simulink model "usrp_fm_amfm"  (R2014b)
settings: Solver=ode45  StartTime=0.0  StopTime=inf  RelTol=1e-3
PreLoadFcn:
  | %%%%%%%%%%%%%%%%%%%%%%%%%%%%%%%%%%%%%%%%%%%%%%%%%%%%%%%%%%%%%%%%%%%%%%%%%%%
  | % check to see if Simulink library folder is missing from the MATLAB path %
  | %%%%%%%%%%%%%%%%%%%%%%%%%%%%%%%%%%%%%%%%%%%%%%%%%%%%%%%%%%%%%%%%%%%%%%%%%%%
  | if isempty(strfind(path, 'rtlsdr_book_library'))
  | 
  |     % create error window
  |     fig_error = figure(...
  |         'Name', 'Error: RTL-SDR Book Library',...
  |         'Toolbar','none',...
  |         'MenuBar','none',...
  |         'NumberTitle','off',...
  |         'Resize','off',...
  |         'WindowStyle','modal');
  |     fig_error.Position(3) = 600;
  |     fig_error.Position(4) = 150;
  |     fig_axes = axes(...
  |         'Parent',fig_error,...
  |         'Position',[0,0,1,1],...
  |         'visible','off');
  |     % error message
  |     t_title = text(.05,.8,...
  |         'MISSING DIRECTORIES',...
  |         'FontSize',11.5);
  |     t_body = text(.075,.6,...
  |         [{'Simulink cannot find the  \it{<root>}\rm / \it{rtlsdr\_book\_library}\rm  folder in the \it{MATLAB Path}\rm.'},...
  |         {'Please set the MATLAB path following the instructions given in Exercise 2.4.'}],...
  |         'FontSize',10.5);
  |     % buttons
  |     btn_path = uicontrol(...
  |         'Parent',fig_error,...
  |         'String','Set Path Now',...
  |         'FontSize',10,...
  |         'Callback', 'pathtool; close(fig_error);',...
  |         'Position', [fig_error.Position(3)/2-210, 30, 200, 30]);
  |     btn_abort = uicontrol(...
  |         'Parent',fig_error,...
  |         'String','No thanks',...
  |         'FontSize',10,...
  |         'Callback', 'close(fig_error); abort=1;',...
  |         'Position', [fig_error.Position(3)/2+10, 30, 200, 30]);
  | 
  |     % pause to allow user to interact with error box
  |     uiwait(fig_error);
  | 
  |     % abort simulation
  |     try
  |         if abort==1
  |             set_param(gcs, 'SimulationCommand', 'stop');
  |         end
  |     end
  | 
  |     % if user has set path, allow diagram to be updated
  |     if ~exist('abort','var')
  |         % create error window
  |         fig_update = figure(...
  |             'Name', 'Update Diagram',...
  |             'Toolbar','none',...
  |             'MenuBar','none',...
  |             'NumberTitle','off',...
  |             'Resize','off');
  |         fig_update.Position(3) = 400;
  |         fig_update.Position(4) = 120;
  |         fig_axes = axes(...
  |             'Parent',fig_update,...
  |             'Position',[0,0,1,1],...
  |             'visible','off');
  |         % instruction message
  |         t_body = text(.075,.7,...
  |             'Once you have set the path, update the block diagram',...
  |             'FontSize',10.5);
  |         % button
  |         btn_update = uicontrol(...
  |             'Parent',fig_update,...
  |             'String','Update Block Diagram',...
  |             'FontSize',10,...
  |             'Callback', 'set_param(gcs,''SimulationCommand'',''update''); close(gcf)',...
  |             'Position', [fig_update.Position(3)/2-100, 30, 200, 30]);
  |     end
  | 
  |     % clear error components
  |     clear('fig_error','fig_update','fig_axes','t_title','t_body','btn_path','btn_abort','btn_update','abort');
  | 
  | end
  | %%%%%%%%%%%%%%%%%%%%%%%%%%%%%%%%%%%%%%%%%%%%%%%%%%%%%%%%%%%%%%%%%%%%%%%%%%%
undefined symbols (not defined in the file): dfilt, fdesignblkfcn, gcbh, startfcn_spectrum_analyzer
libraries: dspmlti4 x3, dspsrcs4 x2, dspvision x1, dsparch4 x1, rtlsdr_book_library x1, commsdrhw_v2 x1
CloseFcn:
  | closefcn_model
Description:
  | Software, Simulation Examples and Design Exercises Licence Agreement
  | 
  | This license agreement refers to the simulation examples, design exercises and files,
  | and associated software MATLAB and Simulink resources that accompany the book:
  | 
  |      Title: Software Defined Radio using MATLAB & Simulink and the RTL-SDR
  |      Published by Strathclyde Academic Media, 2015
  |      Authored by Robert W. Stewart, Kenneth W. Barlee, Dale S.W. Atkinson,
  |      and Louise H. Crockett
  | 
  | and made available as a download from, www.desktopSDR.com or variously acquired
  | by other means such as via USB storage, cloud storage, disk or any other electronic
  | or optical or magnetic storage mechanism. These files and associated software may
  | be used subject to the terms of agreement of the conditions below:
  | 
  |     Copyright © 2015 Robert W. Stewart, Kenneth W. Barlee, Dale S.W. Atkinson,
  |     and Louise H. Crockett
  |     All rights reserved.
  | 
  | Redistribution and use in source and binary forms, with or without modification, are
  | permitted provided that the following conditions are met:
  | 
  |    1.  Redistributions of source code must retain the above copyright notice, this list of
  |         conditions and the following disclaimer.
  | 
  |    2.  Redistributions in binary form must reproduce the above copyright notice, this
  |         list of conditions and the following disclaimer in the documentation and/or other
  |         materials provided with the distribution.
  | 
  |    3.  Neither the name of the copyright holder nor the names of its contributors may
  |         be used to endorse or promote products derived from this software without
  |         specific prior written permission.
  | 
  |    4.  In all cases, the software is, and all modifications and derivatives of the
  |         software shall be, licensed to you solely for use in conjunction with The
  |         MathWorks, Inc. products and service offerings.
  | 
  | THIS SOFTWARE IS PROVIDED BY THE COPYRIGHT HOLDERS AND CONTRIBUTORS
  | "AS IS" AND ANY EXPRESS OR IMPLIED WARRANTIES, INCLUDING, BUT NOT LIMITED
  | TO, THE IMPLIED WARRANTIES OF MERCHANTABILITY AND FITNESS FOR A
  | PARTICULAR PURPOSE ARE DISCLAIMED. IN NO EVENT SHALL THE COPYRIGHT
  | HOLDER OR CONTRIBUTORS BE LIABLE FOR ANY DIRECT, INDIRECT, INCIDENTAL,
  | SPECIAL, EXEMPLARY, OR CONSEQUENTIAL DAMAGES (INCLUDING, BUT NOT
  | LIMITED TO, PROCUREMENT OF SUBSTITUTE GOODS OR SERVICES; LOSS OF USE,
  | DATA, OR PROFITS; OR BUSINESS INTERRUPTION) HOWEVER CAUSED AND ON ANY
  | THEORY OF LIABILITY, WHETHER IN CONTRACT, STRICT LIABILITY, OR TORT
  | (INCLUDING NEGLIGENCE OR OTHERWISE) ARISING IN ANY WAY OUT OF THE USE
  | OF THIS SOFTWARE, EVEN IF ADVISED OF THE POSSIBILITY OF SUCH DAMAGE.
  | 
  | 
  | Audio Tracks used in Simulations Examples and Design Exercises
  | 
  | The music and vocal files used within the Examples files and software within the book
  | were variously written, arranged, performed, recorded and produced by Garrey Rice,
  | Adam Struth, Jamie Struth, Iain Thistlethwaite and also Marshall Craigmyle who
  | collectively, and individually where appropriate, assert and retain all of their copyright,
  | performance and artistic rights. Permission to use and reproduce this music is
  | granted for all purposes associated with MATLAB and Simulink software and the
  | simulation examples and design exercises files that accompany this book. Requests to
  | use the music for any other purpose should be directed to: info@desktopSDR.com.
  | For information on music track names, full credits, and links to the musicians please
  | refer to www.desktopSDR.com/more/audio.
settings Model: SimulationMode=accelerator  Creator=desktopSDR Team  LastModifiedBy=desktopSDR Team
settings DataIOCC: LimitDataPoints=off  SaveOutput=off  SignalLogging=off  SaveTime=off

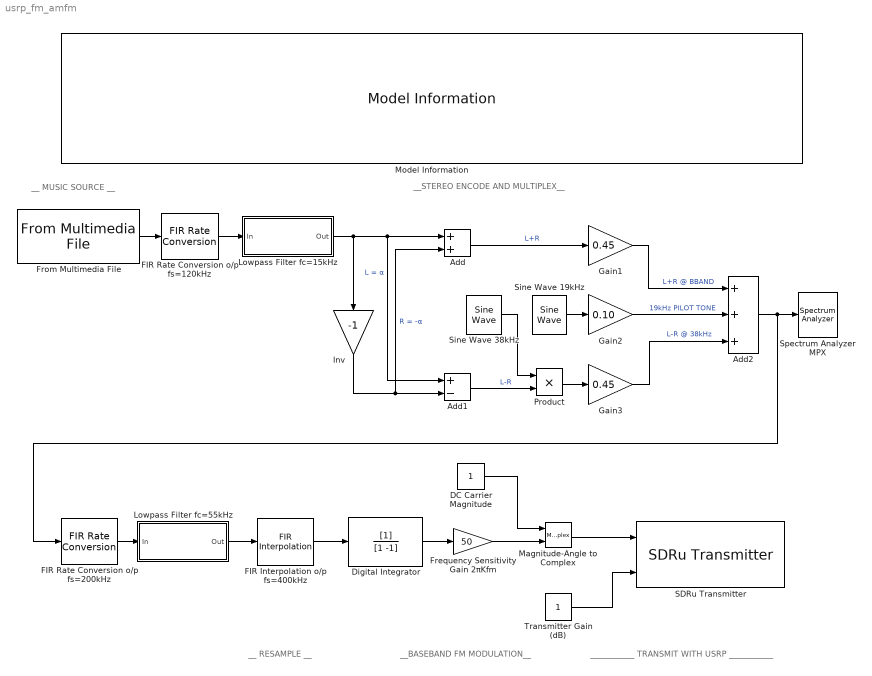
== system usrp_fm_amfm ==
  note: __ MUSIC SOURCE __
  note: __ RESAMPLE __
  note: ___________ TRANSMIT WITH USRP ___________
  note: __BASEBAND FM MODULATION__
  note: __STEREO ENCODE AND MULTIPLEX__
  Add : Sum
  Add1 : Sum  Inputs=+-
  Add2 : Sum  Inputs=+++
  DC Carrier Magnitude : Constant
  Digital Integrator : DiscreteFilter  Denominator=[1 -1]  InputProcessing=Columns as channels (frame based)  FilterStructure=Direct form II transposed  a0EqualsOne=on
  FIR Interpolation o/p fs=400kHz : dspmlti4/FIR Interpolation  h=firpm(100, [0 53e3 65e3 400e3/2]/(400e3/2), [1 1 0 0], [1 1],20)  L=2  framing=Allow multirate processing  outputBufInitCond=0  InputProcessing=Columns as channels (frame based)  firstCoeffDataTypeStr=Inherit: Same word length as input  firstCoeffLastDataTypeStr=Inherit: Same word length as input  firstCoeffMin=[]  firstCoeffMax=[]  outputDataTypeStr=Inherit: Same as accumulator  outputLastDataTypeStr=Inherit: Same as accumulator  outputMin=[]  outputMax=[]  roundingMode=Floor  overflowMode=off  FilterSource=Specify via dialog  FilterObject=Hm_firinterp
  FIR Rate Conversion o/p fs=120kHz : dspmlti4/FIR Rate Conversion  L=5  h=firpm(50, [0 15e3 24e3 240e3/2]/(240e3/2), [1 1 0 0], [1 1],20)  M=2  firstCoeffDataTypeStr=Inherit: Same word length as input  firstCoeffLastDataTypeStr=Inherit: Same word length as input  firstCoeffMin=[]  firstCoeffMax=[]  outputDataTypeStr=Inherit: Same as accumulator  outputLastDataTypeStr=Inherit: Same as accumulator  outputMin=[]  outputMax=[]  roundingMode=Floor  overflowMode=off  FilterSource=Specify via dialog  FilterObject=Hm_firsrc
  FIR Rate Conversion o/p fs=200kHz : dspmlti4/FIR Rate Conversion  L=5  h=firpm(100, [0 53e3 65e3 600e3/2]/(600e3/2), [1 1 0 0], [1 1],20)  M=3  firstCoeffDataTypeStr=Inherit: Same word length as input  firstCoeffLastDataTypeStr=Inherit: Same word length as input  firstCoeffMin=[]  firstCoeffMax=[]  outputDataTypeStr=Inherit: Same as accumulator  outputLastDataTypeStr=Inherit: Same as accumulator  outputMin=[]  outputMax=[]  roundingMode=Floor  overflowMode=off  FilterSource=Specify via dialog  FilterObject=Hm_firsrc
  Frequency Sensitivity Gain 2πKfm : Gain  Gain=50
  From Multimedia File : dspvision/From Multimedia File  inputFilename=../../audio_sources/music2_mono48kHz.wav  loop=on  numPlays=inf  outputStreams=Audio only  videoDataType=single  audioDataType=double  inheritSampleTime=on  userDefinedSampleTime=1/30  noAudioOutput=off  isIntensityVideo=off  fourcc=RGB  colorVideoFormat=One multidimensional signal  outputEOF=off  dataOrg=Column-major  audioFrameSize=600  computeAudioFrameSize=off  outSamplingMode=Sample based
  Gain1 : Gain  Gain=0.45
  Gain2 : Gain  Gain=0.10
  Gain3 : Gain  Gain=0.45
  Inv : Gain  Gain=-1
  Lowpass Filter fc=15kHz : Subsystem  DialogController=fdesignblkfcn  InitFcn=fdesignblkfcn(gcbh, {'InitFcn'});  mask(Lowpass Filter){}
      mask help: Design a lowpass filter
      settings: CopyFcn=fdesignblkfcn(gcbh, {'CopyFcn'});
      mask Help: helpview(mapfilelocation('dsp'), 'dsplowpassfilter');
      mask Display: disp('Lowpass')
  Lowpass Filter fc=55kHz : Subsystem  DialogController=fdesignblkfcn  InitFcn=fdesignblkfcn(gcbh, {'InitFcn'});  mask(Lowpass Filter){}
      mask help: Design a lowpass filter
      settings: CopyFcn=fdesignblkfcn(gcbh, {'CopyFcn'});
      mask Help: helpview(mapfilelocation('dsp'), 'dsplowpassfilter');
      mask Display: disp('Lowpass')
  Magnitude-Angle to Complex : MagnitudeAngleToComplex
  Model Information : rtlsdr_book_library/Additional Tools/Model Information/Model Information
  Product : Product
  SDRu Transmitter : commsdrhw_v2/SDRu Transmitter  rxtx=tx  platform=N200/N210/USRP2  USRP2_IP='169.254.10.2'  USRP_IP_X300='192.168.10.2'  USRP_IP_X310='192.168.10.2'  USRP_serialNumB200=''  USRP_serialNumB210=''  centerFrequency=433.9e6  centerFrequencySrc=Dialog  loOffset=250e3  loOffsetSrc=Dialog  masterClkRateB200=32e6  masterClkRateB210=32e6  masterClkRateX300=200e6  masterClkRateX310=200e6  masterClkRateParam=100e6  gain=10  gainSrc=Input port  decimInterp=250  decimInterpSrc=Dialog  USRP2_IP_NUM=[49 54 57 46 50 53 52 46 49 48 46 50]  frameLength=362  outputDatatype=int16  overrunUnderrunPort=off  sampleTime=1  dboardInfo=|  HOST_DATA_PORT=30000  HOST_CONTROL_PORT=30001  USRP2_DATA_PORT=32769  USRP2_CONTROL_PORT=32768  bufferMode=Continuous streaming  EnableBurstMode=off  NumFramesInBurst=100  USRP_ID='169.254.10.2'
      | dbid: 0
      |           dbName: 'no db found'
      |          freqMin: 0
      |          freqMax: 0
      |          gainMin: 0
      |          gainMax: 0
      |     gainStepSize: 0
  Sine Wave 19kHz : dspsrcs4/Sine Wave  Amplitude=1  Frequency=19e3  Phase=0  SampleMode=Discrete  OutComplex=Real  CompMethod=Trigonometric fcn  TableSize=Speed  SampleTime=1/120e3  SamplesPerFrame=1500  ResetState=Restart at time zero  dataType=double  wordLen=16  udDataType=sfix(16)  fracBitsMode=Best precision  numFracBits=15  OutDataTypeStr=double  LastOutDataTypeStr=double
  Sine Wave 38kHz : dspsrcs4/Sine Wave  Amplitude=1  Frequency=38e3  Phase=0  SampleMode=Discrete  OutComplex=Real  CompMethod=Trigonometric fcn  TableSize=Speed  SampleTime=1/120e3  SamplesPerFrame=1500  ResetState=Restart at time zero  dataType=double  wordLen=16  udDataType=sfix(16)  fracBitsMode=Best precision  numFracBits=15  OutDataTypeStr=double  LastOutDataTypeStr=double
  Spectrum Analyzer MPX : SpectrumAnalyzer  StartFcn=startfcn_spectrum_analyzer;
  Transmitter Gain (dB) : Constant
  wires:
  Digital Integrator/1 -> Frequency Sensitivity Gain 2πKfm/1
  DC Carrier Magnitude/1 -> Magnitude-Angle to Complex/1
  Frequency Sensitivity Gain 2πKfm/1 -> Magnitude-Angle to Complex/2
  FIR Rate Conversion o/p fs=200kHz/1 -> Lowpass Filter fc=55kHz/1(In)
  Lowpass Filter fc=55kHz/1(Out) -> FIR Interpolation o/p fs=400kHz/1
  From Multimedia File/1 -> FIR Rate Conversion o/p fs=120kHz/1
  Magnitude-Angle to Complex/1 -> SDRu Transmitter/1
  Transmitter Gain (dB)/1 -> SDRu Transmitter/2
  FIR Interpolation o/p fs=400kHz/1 -> Digital Integrator/1
  FIR Rate Conversion o/p fs=120kHz/1 -> Lowpass Filter fc=15kHz/1(In)
  Add/1 -> Gain1/1  "L+R"
  Add1/1 -> Product/2  "L-R"
  Gain1/1 -> Add2/1  "L+R @ BBAND"
  Inv/1 -> Add1/2, Add/2  "R = -α"
  Lowpass Filter fc=15kHz/1(Out) -> Inv/1, Add/1, Add1/1  "L = α"
  Sine Wave 38kHz/1 -> Product/1
  Product/1 -> Gain3/1
  Sine Wave 19kHz/1 -> Gain2/1
  Gain2/1 -> Add2/2  "19kHz PILOT TONE"
  Gain3/1 -> Add2/3  "L-R @ 38kHz"
  Add2/1 -> Spectrum Analyzer MPX/1, FIR Rate Conversion o/p fs=200kHz/1

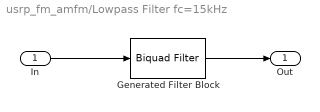
== system usrp_fm_amfm/Lowpass Filter fc=15kHz ==
  In : Inport
  Generated Filter Block : dsparch4/Biquad Filter  Tag=BlockMethodSubSystem  IIRFiltStruct=Direct form II  CoeffSource=Specify via dialog  BiQuadCoeffs=[0.47317005345169666 -0.30307728548160168 0.3552862054548247 1 -1.3238737006712475 0.86511185339799446;0.25407991836614779 0.013136135916053305 0.00082836158684250797 1 -1.5734734560410242 0.70525008464109618;0.26098132032063748 -0.29548649035134594 0.034572981551380208 1 -1.3156763282103388 0.66891715813083463;0.030797704742965809 -0.0062470044848620589 0.0024961066929451189 1 -1.3942015618174157 0.77798854949818474;1.5211188179161075 -2 1.5075788908074403 1 -1.3865253012495609 0.98071245573948018;-0.86987276178120643 0.55655777437114651 -0.25149509973734757 1 -1.357338185996994 0.84525618519026846;0.25557566805887638 0.14108303077480563 0.19172424260597029 1 -1.6306553480127399 0.68783931627099504;0.1592819381000054 0.076004983723057917 0.0061187770260567554 1 -1.8253479266443986 0.82545247207677486;0.07934261365834086 -0.0022173795904536437 0.045369159306579282 1 -1.4840124255643086 0.72683648922007227;1.6187100875684302 -2 1.5743866150788544 1 -1.3664078844337517 0.93151058917172236]  a0Flag=Warning  IC=0  ICnum=0  ICden=0  InputProcessing=Columns as channels (frame based)  denAccumFracLength=30  denProdOutputFracLength=30  secondMemoryFracLength=15  roundingMode=Floor  overflowMode=off  ScaleValues=[0.094760439304554744;1;1;1;1;1;1;1;1;1;3.8950302415849745]  optimizeScaleValues=off  ScaleValueMode=Specify via input port (g)  scaleValueFracLength=14  FilterSource=Specify via dialog  dfiltObjectName=dfilt.df2tsos([1 0.3 0.4],[1 0.1 0.2])
  Out : Outport
  wires:
  In/1 -> Generated Filter Block/1
  Generated Filter Block/1 -> Out/1

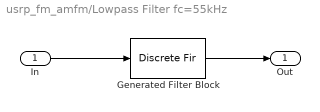
== system usrp_fm_amfm/Lowpass Filter fc=55kHz ==
  In : Inport
  Generated Filter Block : DiscreteFir  Tag=BlockMethodSubSystem  Coefficients=[-6.228788804934224e-06 -6.2062747942014939e-05 4.4773382033788142e-05 5.9223440449491947e-05 -0.00012902946020640376 3.6983343869436008e-07 0.00021622955802696195 -0.00016931108722936932 -0.0002103307922296076 0.0004203176914546472 -4.951070473338399e-07 -0.00061945455119501375 0.00045955373668531705 0.00054592336203957033 -0.0010451333571811132 5.7875515594737832e-07 0.0014336479231852669 -0.0010301309632501858 -0.0011902058631939197 0.0022179757180349115 -5.4654893135257685e-07 -0.0029036740970725563 0.0020428558483851765 0.0023165245463852937 -0.0042401205348852082 3.9622561535849608e-07 0.0053811500338701275 -0.0037343170525407283 -0.0041841946727133456 0.00757496839686401 -1.8393767439645872e-07 -0.009447038967959797 0.0065128999771686211 0.0072630306612990834 -0.013107967803677682 -8.6187196458905747e-08 0.016351486195946893 -0.011316727849119357 -0.012709816490706774 0.023186540784212503 3.6660766273777895e-07 -0.030003289029009606 0.021369917058443037 0.024947578295831729 -0.047965080163758965 -5.4389954901419886e-07 0.074002463452510645 -0.061583217473329108 -0.093026315714072341 0.30230652367204658 0.60000061092233026 0.30230652367204658 -0.093026315714072341 -0.061583217473329108 0.074002463452510645 -5.4389954901419886e-07 -0.047965080163758965 0.024947578295831729 0.021369917058443037 -0.030003289029009606 3.6660766273777895e-07 0.023186540784212503 -0.012709816490706774 -0.011316727849119357 0.016351486195946893 -8.6187196458905747e-08 -0.013107967803677682 0.0072630306612990834 0.0065128999771686211 -0.009447038967959797 -1.8393767439645872e-07 0.00757496839686401 -0.0041841946727133456 -0.0037343170525407283 0.0053811500338701275 3.9622561535849608e-07 -0.0042401205348852082 0.0023165245463852937 0.0020428558483851765 -0.0029036740970725563 -5.4654893135257685e-07 0.0022179757180349115 -0.0011902058631939197 -0.0010301309632501858 0.0014336479231852669 5.7875515594737832e-07 -0.0010451333571811132 0.00054592336203957033 0.00045955373668531705 -0.00061945455119501375 -4.951070473338399e-07 0.0004203176914546472 -0.0002103307922296076 -0.00016931108722936932 0.00021622955802696195 3.6983343869436008e-07 -0.00012902946020640376 5.9223440449491947e-05 4.4773382033788142e-05 -6.2062747942014939e-05 -6.228788804934224e-06]  InputProcessing=Columns as channels (frame based)
  Out : Outport
  wires:
  Generated Filter Block/1 -> Out/1
  In/1 -> Generated Filter Block/1
